simulink library "PosLib"  (R2021a)
settings: Solver=VariableStepAuto  StartTime=0.0  StopTime=10.0  RelTol=1e-3
values from neighbouring files (symbols this model uses):
  clientID = vrep.simxStart('127.0.0.1', port, true, true, 5000, 5)    [InitSim.m]
  vrep = remApi('remoteApi')    [InitSim.m]
libraries: roblocks x5
settings Model: Creator=Harry  LastModifiedBy=Harry

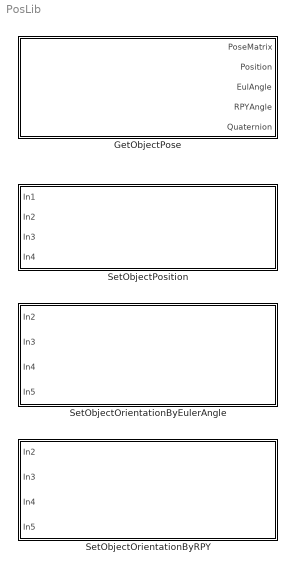
== system PosLib ==
  GetObjectPose : Subsystem  AncestorBlock=PosLib/GetObjectPosition  mask{object_name='L1', relative_object_name='world'}
      mask prompts: object_name "Object name:"; relative_object_name "Relative name:"
      mask DialogControl DescGroupVar Prompt: Instructions
      mask DialogControl DescTextVar Prompt: Relative Object: 'world' means relative to world frame, 'parent' means  relative to parent frame, and you can input other object name.
      mask Display:
      | port_label('output',1,'pose matrix(4*4)')
      | port_label('output',2,'position(x,y,z)')
      | port_label('output',3,'euler angle(ZYZ)')
      | port_label('output',4,'RPY angle(XYZ)')
      | port_label('output',5,'Quaternion')
      | 
      | if ischar(object_name)
      |     color('black');
      |     x=sprintf('GetObjectPose\n\n(%s relative to %s)',object_name,relative_object_name);
      |     disp(x);
      | else
      |     color('red');
      |     disp('Input Error');
      | end
  SetObjectOrientationByEulerAngle : Subsystem  mask{object_name='L2', relative_object_name='world', is_use_vector=on}
      mask prompts: object_name "Object name:"; relative_object_name "Relative frame:"; is_use_vector "Use vector:"
      mask Display:
      | port_label('input',1,'Euler angle(ZYZ)')
      | port_label('input',2,'φ')
      | port_label('input',3,'θ')
      | port_label('input',4,'ψ')
      | 
      | if ischar(object_name)
      |     color('black');
      |     x=sprintf('SetObjectOrientationByEulerAngle\n\n(%s relative to %s)',object_name,relative_object_name);
      |     disp(x);
      | else
      |     color('red');
      |     disp('Input Error');
      | end
      | 
      | color('blue')
      | text(30,8,'Absolute')
  SetObjectOrientationByRPY : Subsystem  mask{object_name='L2', relative_object_name='world', is_use_vector=on}
      mask prompts: object_name "Object name:"; relative_object_name "Relative frame:"; is_use_vector "Use vector:"
      mask Display:
      | port_label('input',1,'RPY angle(XYZ)')
      | port_label('input',2,'roll')
      | port_label('input',3,'pitch')
      | port_label('input',4,'yaw')
      | 
      | if ischar(object_name)
      |     color('black');
      |     x=sprintf('SetObjectOrientationByRPY Rx(y)*Rx(p)*Rx(r)\n\n(%s relative to %s)',object_name,relative_object_name);
      |     disp(x);
      | else
      |     color('red');
      |     disp('Input Error');
      | end
      | 
      | color('blue')
      | text(30,8,'Absolute')
  SetObjectPosition : Subsystem  AncestorBlock=PosLib/GetObjectPosition  mask{object_name='L1', relative_object_name='world', isUseVector=off}
      mask prompts: object_name "Object name:"; relative_object_name "Relative name:"; isUseVector "is use vector:"
      mask DialogControl DescGroupVar Prompt: Instructions
      mask DialogControl DescTextVar Prompt: Relative Object: 'world' means relative to world frame, 'parent' means  relative to parent frame, and you can input other object name.
      mask Display:
      | port_label('input',1,'vector(x,y,z)')
      | port_label('input',2,'x')
      | port_label('input',3,'y')
      | port_label('input',4,'z')
      | 
      | if ischar(object_name)
      |     color('black');
      |     x=sprintf('SetObjectPosition\n(%s relative to %s)',object_name,relative_object_name);
      |     disp(x);
      | else
      |     color('red');
      |     disp('Input Error');
      | end
      | 
      | color('blue')
      | text(15,8,'x,y,z position')

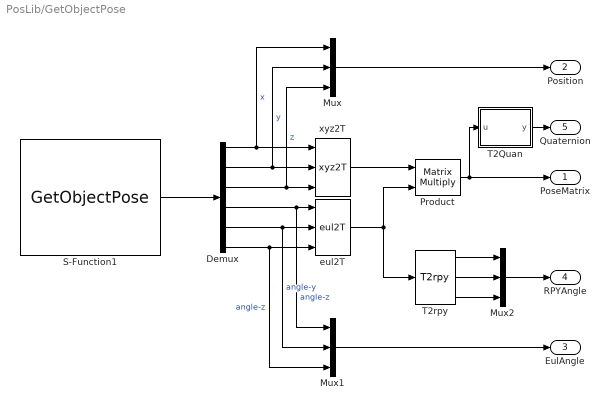
== system PosLib/GetObjectPose ==
  Demux : Demux  Outputs=6
  Mux : Mux  Inputs=3
  Mux1 : Mux  Inputs=3
  Mux2 : Mux  Inputs=3
  Product : Product  Multiplication=Matrix(*)
  S-Function1 : S-Function  FunctionName=GetObjectPose  Parameters=vrep,clientID,object_name,relative_object_name  SFunctionDeploymentMode=off  EnableBusSupport=off
  T2Quan : MATLAB Function  TreatAsAtomicUnit=on
  T2rpy : roblocks/Toolbox/T2rpy  sequence=ZYX  degrees=off
      settings: SourceProductName=roblocks
  eul2T : roblocks/Toolbox/eul2T  degrees=off
      settings: SourceProductName=roblocks
  xyz2T : roblocks/Toolbox/xyz2T
      settings: SourceProductName=roblocks
  PoseMatrix : Outport
  Position : Outport  Port=2
  EulAngle : Outport  Port=3
  RPYAngle : Outport  Port=4
  Quaternion : Outport  Port=5
  wires:
  S-Function1/1 -> Demux/1
  Demux/1 -> Mux/1, xyz2T/1  "x"
  Demux/2 -> Mux/2, xyz2T/2  "y"
  Demux/3 -> Mux/3, xyz2T/3  "z"
  Demux/4 -> Mux1/1, eul2T/1  "angle-z"
  Demux/5 -> Mux1/2, eul2T/2  "angle-y"
  Demux/6 -> Mux1/3, eul2T/3  "angle-z"
  xyz2T/1 -> Product/1
  eul2T/1 -> T2rpy/1, Product/2
  Product/1 -> T2Quan/1(u), PoseMatrix/1
  Mux/1 -> Position/1
  Mux1/1 -> EulAngle/1
  T2rpy/1 -> Mux2/1
  T2rpy/2 -> Mux2/2
  T2rpy/3 -> Mux2/3
  Mux2/1 -> RPYAngle/1
  T2Quan/1(y) -> Quaternion/1

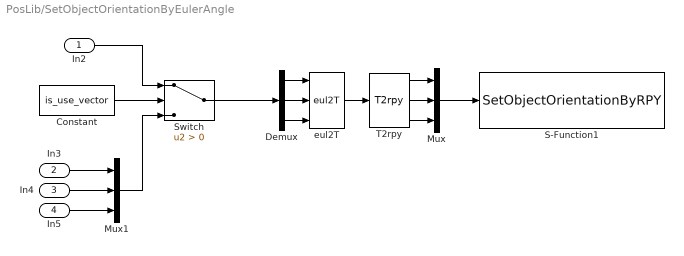
== system PosLib/SetObjectOrientationByEulerAngle ==
  In2 : Inport
  In3 : Inport  Port=2
  In4 : Inport  Port=3
  In5 : Inport  Port=4
  Constant : Constant  Value=is_use_vector
  Demux : Demux  Outputs=3
  Mux : Mux  Inputs=3
  Mux1 : Mux  Inputs=3
  S-Function1 : S-Function  FunctionName=SetObjectOrientationByRPY  Parameters=vrep,clientID,object_name,relative_object_name  SFunctionDeploymentMode=off  EnableBusSupport=off
  Switch : Switch  Criteria=u2 > Threshold
  T2rpy : roblocks/Toolbox/T2rpy  sequence=ZYX  degrees=off
      settings: SourceProductName=roblocks
  eul2T : roblocks/Toolbox/eul2T  degrees=off
      settings: SourceProductName=roblocks
  wires:
  T2rpy/1 -> Mux/1
  T2rpy/2 -> Mux/2
  T2rpy/3 -> Mux/3
  eul2T/1 -> T2rpy/1
  Demux/1 -> eul2T/1
  Demux/2 -> eul2T/2
  Demux/3 -> eul2T/3
  Mux/1 -> S-Function1/1
  Mux1/1 -> Switch/3
  In4/1 -> Mux1/2
  In2/1 -> Switch/1
  In5/1 -> Mux1/3
  Switch/1 -> Demux/1
  Constant/1 -> Switch/2
  In3/1 -> Mux1/1

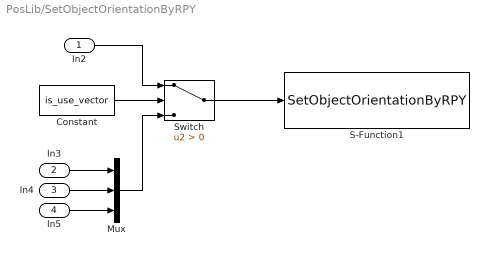
== system PosLib/SetObjectOrientationByRPY ==
  In2 : Inport
  In3 : Inport  Port=2
  In4 : Inport  Port=3
  In5 : Inport  Port=4
  Constant : Constant  Value=is_use_vector
  Mux : Mux  Inputs=3
  S-Function1 : S-Function  FunctionName=SetObjectOrientationByRPY  Parameters=vrep,clientID,object_name,relative_object_name  SFunctionDeploymentMode=off  EnableBusSupport=off
  Switch : Switch  Criteria=u2 > Threshold
  wires:
  Switch/1 -> S-Function1/1
  In2/1 -> Switch/1
  In3/1 -> Mux/1
  In4/1 -> Mux/2
  In5/1 -> Mux/3
  Mux/1 -> Switch/3
  Constant/1 -> Switch/2

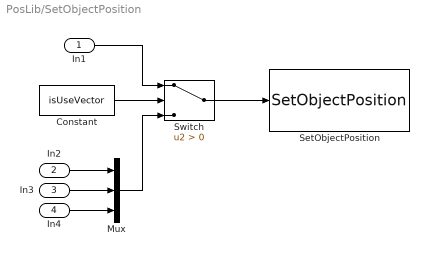
== system PosLib/SetObjectPosition ==
  In1 : Inport
  In2 : Inport  Port=2
  In3 : Inport  Port=3
  In4 : Inport  Port=4
  Constant : Constant  Value=isUseVector
  Mux : Mux  Inputs=3
  SetObjectPosition : S-Function  FunctionName=SetObjectPosition  Parameters=vrep,clientID,object_name,relative_object_name  SFunctionDeploymentMode=off  EnableBusSupport=off
  Switch : Switch  Criteria=u2 > Threshold
  wires:
  In1/1 -> Switch/1
  Switch/1 -> SetObjectPosition/1
  In2/1 -> Mux/1
  In3/1 -> Mux/2
  In4/1 -> Mux/3
  Mux/1 -> Switch/3
  Constant/1 -> Switch/2

== matlab function PosLib/GetObjectPose/T2Quan ==
  data: u input; y output
function y = fcn(u)
    q0 = 0.5*sqrt(1+u(1,1)+u(2,2)+u(3,3));
    q1 = (u(3,2)-u(2,3))/(4*q0);
    q2 = (u(1,3)-u(3,1))/(4*q0);
    q3 = (u(2,1)-u(1,2))/(4*q0);
    y = [q0,q1,q2,q3];
end
